simulink model "RCCA_neliniar_releu"  (R2021a)
settings: Solver=FixedStepAuto  StartTime=0.0  StopTime=20  FixedStep=0.001  RelTol=1e-6
values from neighbouring files (symbols this model uses):
  c0 = 5.4698    [initializare_model.m]
  ci = 10    [initializare_model.m]
  EdR = 49584/8.32    (= 5959.61538462)    [initializare_model.m]
  hA = kT*At    (= 18821.555234)    [initializare_model.m]
  k0 = 34930800    [initializare_model.m]
  mdH = 24953    [initializare_model.m]
  q = 10    [initializare_model.m]
  rcp = 2093    [initializare_model.m]
  T0 = 339.437    [initializare_model.m]
  Ti = 38+273    (= 311)    [initializare_model.m]
  V = 10    [initializare_model.m]
undefined symbols (not defined in the file or in its folder): kreg, tdreg, tireg, tkreg, ttdreg, ttireg
libraries: pid_lib x3
settings Model: Creator=PS  LastModifiedBy=Automatica
settings SolverCC: ZeroCrossAlgorithm=Adaptive  AlgebraicLoopSolver=TrustRegion
settings DataIOCC: ReturnWorkspaceOutputs=off
settings DebuggingCC: IgnoredZcDiagnostic=none  SFMachineParentedDataDiag=warning  ArithmeticOperatorsInVariantConditions=warning
settings SFSimCC: SimUseLocalCustomCode=off  CustomCodeUndefinedFunction=UseInterfaceOnly
settings RTWCC: RTWUseLocalCustomCode=off

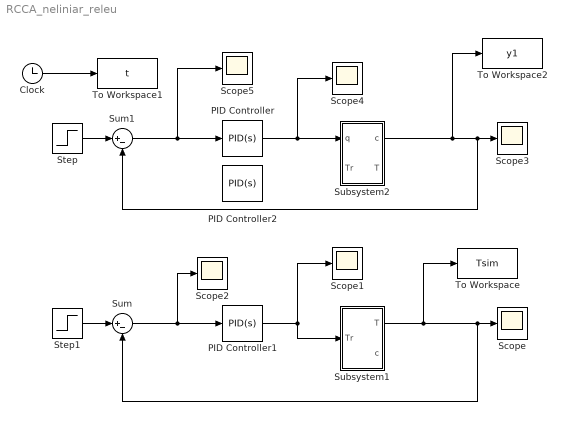
== system RCCA_neliniar_releu ==
  Clock : Clock
  PID Controller : pid_lib/PID Controller  Controller=PID  Form=Parallel  TimeDomain=Continuous-time  UseExternalTs=off  SampleTime=-1  IntegratorMethod=Forward Euler  FilterMethod=Forward Euler  ControllerParametersSource=internal  P=kreg  I=kreg/tireg  D=kreg*tdreg  UseFilter=on  N=100  TunerSelectOption=Transfer Function Based (PID Tuner App)  InitialConditionSource=internal  InitialConditionForIntegrator=q  InitialConditionForFilter=0  DifferentiatorICPrevScaledInput=0  ExternalReset=none  TrackingMode=off  Kt=1  LimitOutput=off  SatLimitsSource=internal  UpperSaturationLimit=inf  LowerSaturationLimit=-inf  LinearizeAsGain=on  AntiWindupMode=none  Kb=1  POutMin=[]  POutMax=[]  IOutMin=[]  IOutMax=[]  DOutMin=[]  DOutMax=[]  NOutMin=[]  NOutMax=[]  SumOutMin=[]  SumOutMax=[]  SaturationOutMin=[]  SaturationOutMax=[]  PParamMin=[]  PParamMax=[]  IParamMin=[]  IParamMax=[]  DParamMin=[]  DParamMax=[]  NParamMin=[]  NParamMax=[]  KbParamMin=[]  KbParamMax=[]  KtParamMin=[]  KtParamMax=[]  KbOutMin=[]  KbOutMax=[]  KtOutMin=[]  KtOutMax=[]  IntegratorOutMin=[]  IntegratorOutMax=[]  FilterOutMin=[]  FilterOutMax=[]  SumI1OutMin=[]  SumI1OutMax=[]  SumI2OutMin=[]  SumI2OutMax=[]  SumI3OutMin=[]  SumI3OutMax=[]  SumI4OutMin=[]  SumI4OutMax=[]  SumDOutMin=[]  SumDOutMax=[]  DifferentiatorOutMin=[]  DifferentiatorOutMax=[]  FilterDiffOutCoefMin=[]  FilterDiffOutCoefMax=[]  ReciprocalOutMin=[]  ReciprocalOutMax=[]  SumDenOutMin=[]  SumDenOutMax=[]  SumNumOutMin=[]  SumNumOutMax=[]  DivideOutMin=[]  DivideOutMax=[]  UdiffTsProdOutMin=[]  UdiffTsProdOutMax=[]  NTsProdOutMin=[]  NTsProdOutMax=[]  UintegralTsProdOutMin=[]  UintegralTsProdOutMax=[]  UngainTsProdOutMin=[]  UngainTsProdOutMax=[]  IntegratorContinuousStateAttributes=''  IntegratorStateMustResolveToSignalObject=off  IntegratorRTWStateStorageClass=Auto  FilterContinuousStateAttributes=''  FilterStateMustResolveToSignalObject=off  FilterRTWStateStorageClass=Auto  ParallelPVariant=InternalParameters  IdealPVariant=Disabled  IVariant=InternalParameters  DVariant=InternalParameters  IntegratorVariant=Continuous  SatVariant=Disabled  AWVariant=Passthrough  PCopyVariant=Disabled  TRVariant=Disabled  FdbkBlocksVariant=Forward  IdealPFdbkVariant=Disabled  SatFdbkVariant=Disabled  DerivativeFilterVariant=ContFilter  NVariant=InternalParameters  NCopyVariant=Disabled  FilterICVariant=InternalICsFilter  IntegratorICVariant=InternalICs  ExternalResetVariant=Disabled  TRSumVariant=Passthrough  SumFdbkVariant=Disabled  SumVariant=Sum_PID  TsampFilterVariant=InternalTs  TsampNgainVariant=Passthrough  TsampIntegralVariant=Passthrough  ExternalSaturationOutDataTypeStr=Inherit: Same as second input
  PID Controller1 : pid_lib/PID Controller  Controller=PID  Form=Parallel  TimeDomain=Continuous-time  UseExternalTs=off  SampleTime=-1  IntegratorMethod=Forward Euler  FilterMethod=Forward Euler  ControllerParametersSource=internal  P=tkreg  I=tkreg/ttireg  D=tkreg*ttdreg  UseFilter=on  N=100  TunerSelectOption=Transfer Function Based (PID Tuner App)  InitialConditionSource=internal  InitialConditionForIntegrator=Tr  InitialConditionForFilter=0  DifferentiatorICPrevScaledInput=0  ExternalReset=none  TrackingMode=off  Kt=1  LimitOutput=off  SatLimitsSource=internal  UpperSaturationLimit=inf  LowerSaturationLimit=-inf  LinearizeAsGain=on  AntiWindupMode=none  Kb=1  POutMin=[]  POutMax=[]  IOutMin=[]  IOutMax=[]  DOutMin=[]  DOutMax=[]  NOutMin=[]  NOutMax=[]  SumOutMin=[]  SumOutMax=[]  SaturationOutMin=[]  SaturationOutMax=[]  PParamMin=[]  PParamMax=[]  IParamMin=[]  IParamMax=[]  DParamMin=[]  DParamMax=[]  NParamMin=[]  NParamMax=[]  KbParamMin=[]  KbParamMax=[]  KtParamMin=[]  KtParamMax=[]  KbOutMin=[]  KbOutMax=[]  KtOutMin=[]  KtOutMax=[]  IntegratorOutMin=[]  IntegratorOutMax=[]  FilterOutMin=[]  FilterOutMax=[]  SumI1OutMin=[]  SumI1OutMax=[]  SumI2OutMin=[]  SumI2OutMax=[]  SumI3OutMin=[]  SumI3OutMax=[]  SumI4OutMin=[]  SumI4OutMax=[]  SumDOutMin=[]  SumDOutMax=[]  DifferentiatorOutMin=[]  DifferentiatorOutMax=[]  FilterDiffOutCoefMin=[]  FilterDiffOutCoefMax=[]  ReciprocalOutMin=[]  ReciprocalOutMax=[]  SumDenOutMin=[]  SumDenOutMax=[]  SumNumOutMin=[]  SumNumOutMax=[]  DivideOutMin=[]  DivideOutMax=[]  UdiffTsProdOutMin=[]  UdiffTsProdOutMax=[]  NTsProdOutMin=[]  NTsProdOutMax=[]  UintegralTsProdOutMin=[]  UintegralTsProdOutMax=[]  UngainTsProdOutMin=[]  UngainTsProdOutMax=[]  IntegratorContinuousStateAttributes=''  IntegratorStateMustResolveToSignalObject=off  IntegratorRTWStateStorageClass=Auto  FilterContinuousStateAttributes=''  FilterStateMustResolveToSignalObject=off  FilterRTWStateStorageClass=Auto  ParallelPVariant=InternalParameters  IdealPVariant=Disabled  IVariant=InternalParameters  DVariant=InternalParameters  IntegratorVariant=Continuous  SatVariant=Disabled  AWVariant=Passthrough  PCopyVariant=Disabled  TRVariant=Disabled  FdbkBlocksVariant=Forward  IdealPFdbkVariant=Disabled  SatFdbkVariant=Disabled  DerivativeFilterVariant=ContFilter  NVariant=InternalParameters  NCopyVariant=Disabled  FilterICVariant=InternalICsFilter  IntegratorICVariant=InternalICs  ExternalResetVariant=Disabled  TRSumVariant=Passthrough  SumFdbkVariant=Disabled  SumVariant=Sum_PID  TsampFilterVariant=InternalTs  TsampNgainVariant=Passthrough  TsampIntegralVariant=Passthrough  ExternalSaturationOutDataTypeStr=Inherit: Same as second input
  PID Controller2 : pid_lib/PID Controller  Controller=PID  Form=Parallel  TimeDomain=Continuous-time  UseExternalTs=off  SampleTime=-1  IntegratorMethod=Forward Euler  FilterMethod=Forward Euler  ControllerParametersSource=internal  P=tkreg  I=tkreg/ttireg  D=tkreg*ttdreg  UseFilter=on  N=100  TunerSelectOption=Transfer Function Based (PID Tuner App)  InitialConditionSource=internal  InitialConditionForIntegrator=Tr  InitialConditionForFilter=0  DifferentiatorICPrevScaledInput=0  ExternalReset=none  TrackingMode=off  Kt=1  LimitOutput=off  SatLimitsSource=internal  UpperSaturationLimit=inf  LowerSaturationLimit=-inf  LinearizeAsGain=on  AntiWindupMode=none  Kb=1  POutMin=[]  POutMax=[]  IOutMin=[]  IOutMax=[]  DOutMin=[]  DOutMax=[]  NOutMin=[]  NOutMax=[]  SumOutMin=[]  SumOutMax=[]  SaturationOutMin=[]  SaturationOutMax=[]  PParamMin=[]  PParamMax=[]  IParamMin=[]  IParamMax=[]  DParamMin=[]  DParamMax=[]  NParamMin=[]  NParamMax=[]  KbParamMin=[]  KbParamMax=[]  KtParamMin=[]  KtParamMax=[]  KbOutMin=[]  KbOutMax=[]  KtOutMin=[]  KtOutMax=[]  IntegratorOutMin=[]  IntegratorOutMax=[]  FilterOutMin=[]  FilterOutMax=[]  SumI1OutMin=[]  SumI1OutMax=[]  SumI2OutMin=[]  SumI2OutMax=[]  SumI3OutMin=[]  SumI3OutMax=[]  SumI4OutMin=[]  SumI4OutMax=[]  SumDOutMin=[]  SumDOutMax=[]  DifferentiatorOutMin=[]  DifferentiatorOutMax=[]  FilterDiffOutCoefMin=[]  FilterDiffOutCoefMax=[]  ReciprocalOutMin=[]  ReciprocalOutMax=[]  SumDenOutMin=[]  SumDenOutMax=[]  SumNumOutMin=[]  SumNumOutMax=[]  DivideOutMin=[]  DivideOutMax=[]  UdiffTsProdOutMin=[]  UdiffTsProdOutMax=[]  NTsProdOutMin=[]  NTsProdOutMax=[]  UintegralTsProdOutMin=[]  UintegralTsProdOutMax=[]  UngainTsProdOutMin=[]  UngainTsProdOutMax=[]  IntegratorContinuousStateAttributes=''  IntegratorStateMustResolveToSignalObject=off  IntegratorRTWStateStorageClass=Auto  FilterContinuousStateAttributes=''  FilterStateMustResolveToSignalObject=off  FilterRTWStateStorageClass=Auto  ParallelPVariant=InternalParameters  IdealPVariant=Disabled  IVariant=InternalParameters  DVariant=InternalParameters  IntegratorVariant=Continuous  SatVariant=Disabled  AWVariant=Passthrough  PCopyVariant=Disabled  TRVariant=Disabled  FdbkBlocksVariant=Forward  IdealPFdbkVariant=Disabled  SatFdbkVariant=Disabled  DerivativeFilterVariant=ContFilter  NVariant=InternalParameters  NCopyVariant=Disabled  FilterICVariant=InternalICsFilter  IntegratorICVariant=InternalICs  ExternalResetVariant=Disabled  TRSumVariant=Passthrough  SumFdbkVariant=Disabled  SumVariant=Sum_PID  TsampFilterVariant=InternalTs  TsampNgainVariant=Passthrough  TsampIntegralVariant=Passthrough  ExternalSaturationOutDataTypeStr=Inherit: Same as second input
  Scope{,1..5} (6 alike) : Scope
  Step : Step  Time=0  Before=c0  After=c0+0.1  SampleTime=0
  Step1 : Step  Time=0  Before=c0  After=c0+0.1  SampleTime=0
  Subsystem1 : Subsystem
  Subsystem2 : Subsystem
  Sum : Sum  Inputs=|+-  InputSameDT=on  SaturateOnIntegerOverflow=on  OutDataTypeStr=Inherit: Same as first input
  Sum1 : Sum  Inputs=|+-  InputSameDT=on  SaturateOnIntegerOverflow=on  OutDataTypeStr=Inherit: Same as first input
  To Workspace : ToWorkspace  VariableName=Tsim  SampleTime=-1
  To Workspace1 : ToWorkspace  VariableName=t  SampleTime=-1
  To Workspace2 : ToWorkspace  VariableName=y1  SampleTime=-1
  wires:
  Sum/1 -> PID Controller1/1, Scope2/1
  Step1/1 -> Sum/1
  Clock/1 -> To Workspace1/1
  Subsystem1/1("T   ") -> Scope/1, Sum/2, To Workspace/1
  Subsystem2/1(c) -> Scope3/1, Sum1/2, To Workspace2/1
  Sum1/1 -> PID Controller/1, Scope5/1
  Step/1 -> Sum1/1
  PID Controller/1 -> Scope4/1, Subsystem2/1(q)
  PID Controller1/1 -> Scope1/1, Subsystem1/1(Tr)

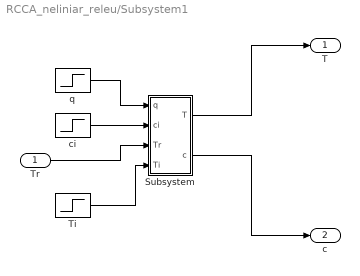
== system RCCA_neliniar_releu/Subsystem1 ==
  Tr : Inport
  Subsystem : Subsystem
  Ti : Step  Time=0  Before=Ti  After=Ti  SampleTime=0
  ci : Step  Time=0  Before=ci  After=ci  SampleTime=0
  "q  " : Step  Time=0  Before=q  After=q  SampleTime=0
  "T   " : Outport
  "c     " : Outport  Port=2
  wires:
  "q  "/1 -> Subsystem/1(q)
  ci/1 -> Subsystem/2(ci)
  Ti/1 -> Subsystem/4(Ti)
  Tr/1 -> Subsystem/3(Tr)
  Subsystem/2("c   ") -> "c     "/1
  Subsystem/1("T  ") -> "T   "/1

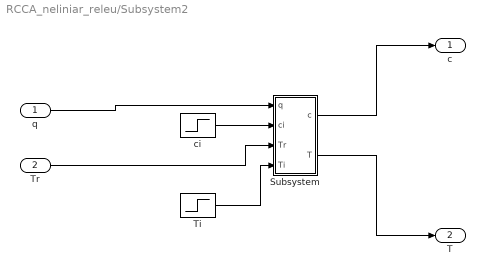
== system RCCA_neliniar_releu/Subsystem2 ==
  q : Inport
  Tr : Inport  Port=2
  Subsystem : Subsystem
  Ti : Step  Time=0  Before=Ti  After=Ti  SampleTime=0
  ci : Step  Time=0  Before=ci  After=ci  SampleTime=0
  c : Outport
  "T  " : Outport  Port=2
  wires:
  q/1 -> Subsystem/1(q)
  ci/1 -> Subsystem/2(ci)
  Ti/1 -> Subsystem/4(Ti)
  Tr/1 -> Subsystem/3(Tr)
  Subsystem/2("T  ") -> "T  "/1
  Subsystem/1(c) -> c/1

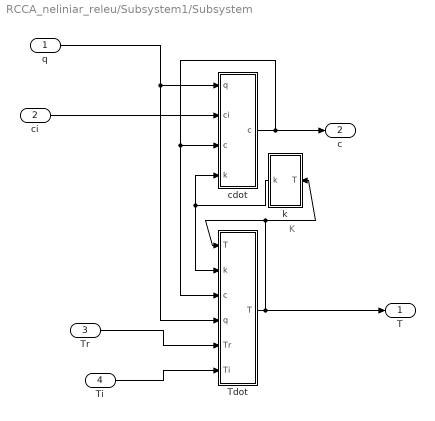
== system RCCA_neliniar_releu/Subsystem1/Subsystem ==
  note: K
  q : Inport
  ci : Inport  Port=2
  Tr : Inport  Port=3
  Ti : Inport  Port=4
  Tdot : Subsystem
  cdot : Subsystem
  k : Subsystem
  "T  " : Outport
  "c   " : Outport  Port=2
  wires:
  Tdot/1("T  ") -> "T  "/1, k/1(T), Tdot/1(T)
  k/1(k) -> Tdot/2(k), cdot/4(k)
  cdot/1(c) -> "c   "/1, cdot/3("c  "), Tdot/3(c)
  q/1 -> cdot/1(q), Tdot/4(q)
  Ti/1 -> Tdot/6(Ti)
  ci/1 -> cdot/2(ci)
  Tr/1 -> Tdot/5(Tr)

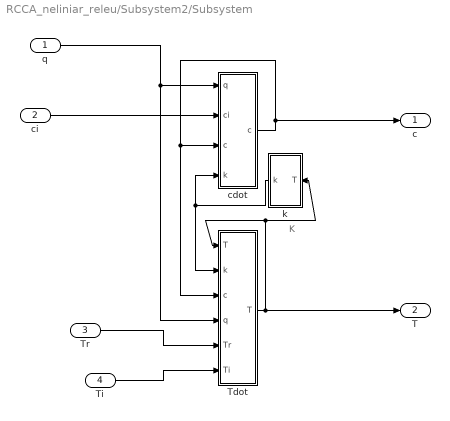
== system RCCA_neliniar_releu/Subsystem2/Subsystem ==
  note: K
  q : Inport
  ci : Inport  Port=2
  Tr : Inport  Port=3
  Ti : Inport  Port=4
  Tdot : Subsystem
  cdot : Subsystem
  k : Subsystem
  c : Outport
  "T  " : Outport  Port=2
  wires:
  Tdot/1("T  ") -> "T  "/1, k/1(T), Tdot/1(T)
  k/1(k) -> Tdot/2(k), cdot/4(k)
  cdot/1(c) -> c/1, cdot/3("c  "), Tdot/3(c)
  q/1 -> cdot/1(q), Tdot/4(q)
  Ti/1 -> Tdot/6(Ti)
  ci/1 -> cdot/2(ci)
  Tr/1 -> Tdot/5(Tr)

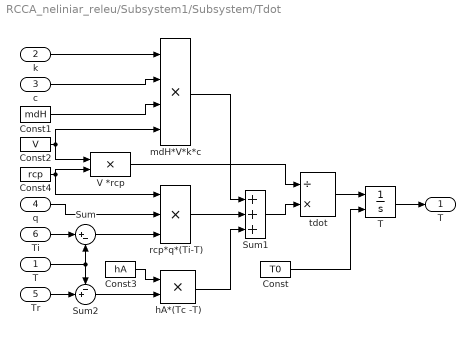
== system RCCA_neliniar_releu/Subsystem1/Subsystem/Tdot ==
  T : Inport  Interpolate=off
  k : Inport  Port=2  Interpolate=off
  c : Inport  Port=3  Interpolate=off
  q : Inport  Port=4  Interpolate=off
  Tr : Inport  Port=5  Interpolate=off
  Ti : Inport  Port=6  Interpolate=off
  Const : Constant  Value=T0
  Const1 : Constant  Value=mdH
  Const2 : Constant  Value=V
  Const3 : Constant  Value=hA
  Const4 : Constant  Value=rcp
  Sum : Sum  Inputs=|+-  InputSameDT=on  SaturateOnIntegerOverflow=on  OutDataTypeStr=Inherit: Same as first input
  Sum1 : Sum  Inputs=+++  InputSameDT=on  SaturateOnIntegerOverflow=on  OutDataTypeStr=Inherit: Same as first input
  Sum2 : Sum  Inputs=-+|  InputSameDT=on  SaturateOnIntegerOverflow=on  OutDataTypeStr=Inherit: Same as first input
  "T " : Integrator  InitialConditionSource=external
  V *rcp : Product  Inputs=**  InputSameDT=on  RndMeth=Zero  SaturateOnIntegerOverflow=on  OutDataTypeStr=Inherit: Same as first input
  hA*(Tc -T) : Product  Inputs=**  InputSameDT=on  RndMeth=Zero  SaturateOnIntegerOverflow=on  OutDataTypeStr=Inherit: Same as first input
  mdH*V*k*c : Product  Inputs=****  InputSameDT=on  RndMeth=Zero  SaturateOnIntegerOverflow=on  OutDataTypeStr=Inherit: Same as first input
  rcp*q*(Ti-T) : Product  Inputs=***  InputSameDT=on  RndMeth=Zero  SaturateOnIntegerOverflow=on  OutDataTypeStr=Inherit: Same as first input
  tdot : Product  Inputs=/*  InputSameDT=on  RndMeth=Zero  SaturateOnIntegerOverflow=on  OutDataTypeStr=Inherit: Same as first input
  "T  " : Outport
  wires:
  Ti/1 -> Sum/1
  Sum/1 -> rcp*q*(Ti-T)/3
  q/1 -> rcp*q*(Ti-T)/2
  T/1 -> Sum/2, Sum2/1
  Tr/1 -> Sum2/2
  Sum2/1 -> hA*(Tc -T)/2
  Const3/1 -> hA*(Tc -T)/1
  k/1 -> mdH*V*k*c/1
  c/1 -> mdH*V*k*c/2
  Const1/1 -> mdH*V*k*c/3
  mdH*V*k*c/1 -> Sum1/1
  rcp*q*(Ti-T)/1 -> Sum1/2
  hA*(Tc -T)/1 -> Sum1/3
  Const2/1 -> mdH*V*k*c/4, V *rcp/1
  Const4/1 -> rcp*q*(Ti-T)/1, V *rcp/2
  V *rcp/1 -> tdot/1
  Sum1/1 -> tdot/2
  tdot/1 -> "T "/1
  Const/1 -> "T "/2
  "T "/1 -> "T  "/1

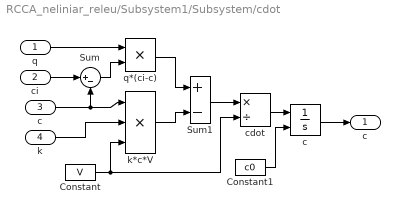
== system RCCA_neliniar_releu/Subsystem1/Subsystem/cdot ==
  q : Inport  Interpolate=off
  ci : Inport  Port=2  Interpolate=off
  "c  " : Inport  Port=3  Interpolate=off
  k : Inport  Port=4  Interpolate=off
  Constant : Constant  Value=V
  Constant1 : Constant  Value=c0
  Sum : Sum  Inputs=|+-  InputSameDT=on  SaturateOnIntegerOverflow=on  OutDataTypeStr=Inherit: Same as first input
  Sum1 : Sum  Inputs=+-  InputSameDT=on  SaturateOnIntegerOverflow=on  OutDataTypeStr=Inherit: Same as first input
  "c " : Integrator  InitialConditionSource=external
  cdot : Product  Inputs=*/  InputSameDT=on  RndMeth=Zero  SaturateOnIntegerOverflow=on  OutDataTypeStr=Inherit: Same as first input
  k*c*V : Product  Inputs=***  InputSameDT=on  RndMeth=Zero  SaturateOnIntegerOverflow=on  OutDataTypeStr=Inherit: Same as first input
  q*(ci-c) : Product  Inputs=**  InputSameDT=on  RndMeth=Zero  SaturateOnIntegerOverflow=on  OutDataTypeStr=Inherit: Same as first input
  c : Outport
  wires:
  ci/1 -> Sum/1
  "c  "/1 -> k*c*V/1, Sum/2
  q/1 -> q*(ci-c)/1
  Sum/1 -> q*(ci-c)/2
  k/1 -> k*c*V/2
  q*(ci-c)/1 -> Sum1/1
  k*c*V/1 -> Sum1/2
  Sum1/1 -> cdot/1
  Constant/1 -> k*c*V/3, cdot/2
  cdot/1 -> "c "/1
  "c "/1 -> c/1
  Constant1/1 -> "c "/2

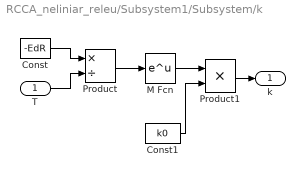
== system RCCA_neliniar_releu/Subsystem1/Subsystem/k ==
  T : Inport  Interpolate=off
  Const : Constant  Value=-EdR
  Const1 : Constant  Value=k0
  M Fcn : Math  SignedPower=on  SaturateOnIntegerOverflow=on
  Product : Product  Inputs=*/  InputSameDT=on  RndMeth=Zero  SaturateOnIntegerOverflow=on  OutDataTypeStr=Inherit: Same as first input
  Product1 : Product  Inputs=**  InputSameDT=on  RndMeth=Zero  SaturateOnIntegerOverflow=on  OutDataTypeStr=Inherit: Same as first input
  k : Outport
  wires:
  Const/1 -> Product/1
  T/1 -> Product/2
  Product/1 -> M Fcn/1
  M Fcn/1 -> Product1/1
  Const1/1 -> Product1/2
  Product1/1 -> k/1

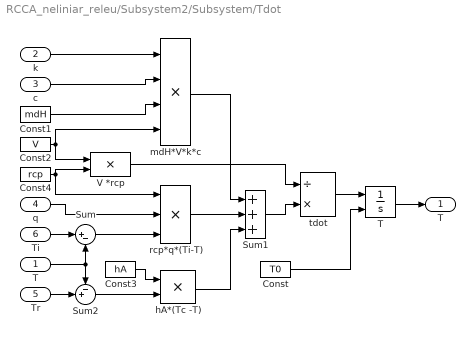
== system RCCA_neliniar_releu/Subsystem2/Subsystem/Tdot ==
  T : Inport  Interpolate=off
  k : Inport  Port=2  Interpolate=off
  c : Inport  Port=3  Interpolate=off
  q : Inport  Port=4  Interpolate=off
  Tr : Inport  Port=5  Interpolate=off
  Ti : Inport  Port=6  Interpolate=off
  Const : Constant  Value=T0
  Const1 : Constant  Value=mdH
  Const2 : Constant  Value=V
  Const3 : Constant  Value=hA
  Const4 : Constant  Value=rcp
  Sum : Sum  Inputs=|+-  InputSameDT=on  SaturateOnIntegerOverflow=on  OutDataTypeStr=Inherit: Same as first input
  Sum1 : Sum  Inputs=+++  InputSameDT=on  SaturateOnIntegerOverflow=on  OutDataTypeStr=Inherit: Same as first input
  Sum2 : Sum  Inputs=-+|  InputSameDT=on  SaturateOnIntegerOverflow=on  OutDataTypeStr=Inherit: Same as first input
  "T " : Integrator  InitialConditionSource=external
  V *rcp : Product  Inputs=**  InputSameDT=on  RndMeth=Zero  SaturateOnIntegerOverflow=on  OutDataTypeStr=Inherit: Same as first input
  hA*(Tc -T) : Product  Inputs=**  InputSameDT=on  RndMeth=Zero  SaturateOnIntegerOverflow=on  OutDataTypeStr=Inherit: Same as first input
  mdH*V*k*c : Product  Inputs=****  InputSameDT=on  RndMeth=Zero  SaturateOnIntegerOverflow=on  OutDataTypeStr=Inherit: Same as first input
  rcp*q*(Ti-T) : Product  Inputs=***  InputSameDT=on  RndMeth=Zero  SaturateOnIntegerOverflow=on  OutDataTypeStr=Inherit: Same as first input
  tdot : Product  Inputs=/*  InputSameDT=on  RndMeth=Zero  SaturateOnIntegerOverflow=on  OutDataTypeStr=Inherit: Same as first input
  "T  " : Outport
  wires:
  Ti/1 -> Sum/1
  Sum/1 -> rcp*q*(Ti-T)/3
  q/1 -> rcp*q*(Ti-T)/2
  T/1 -> Sum/2, Sum2/1
  Tr/1 -> Sum2/2
  Sum2/1 -> hA*(Tc -T)/2
  Const3/1 -> hA*(Tc -T)/1
  k/1 -> mdH*V*k*c/1
  c/1 -> mdH*V*k*c/2
  Const1/1 -> mdH*V*k*c/3
  mdH*V*k*c/1 -> Sum1/1
  rcp*q*(Ti-T)/1 -> Sum1/2
  hA*(Tc -T)/1 -> Sum1/3
  Const2/1 -> mdH*V*k*c/4, V *rcp/1
  Const4/1 -> rcp*q*(Ti-T)/1, V *rcp/2
  V *rcp/1 -> tdot/1
  Sum1/1 -> tdot/2
  tdot/1 -> "T "/1
  Const/1 -> "T "/2
  "T "/1 -> "T  "/1

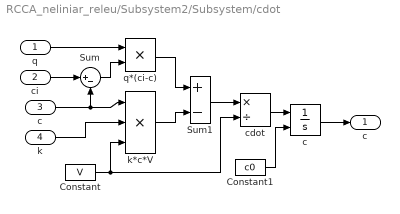
== system RCCA_neliniar_releu/Subsystem2/Subsystem/cdot ==
  q : Inport  Interpolate=off
  ci : Inport  Port=2  Interpolate=off
  "c  " : Inport  Port=3  Interpolate=off
  k : Inport  Port=4  Interpolate=off
  Constant : Constant  Value=V
  Constant1 : Constant  Value=c0
  Sum : Sum  Inputs=|+-  InputSameDT=on  SaturateOnIntegerOverflow=on  OutDataTypeStr=Inherit: Same as first input
  Sum1 : Sum  Inputs=+-  InputSameDT=on  SaturateOnIntegerOverflow=on  OutDataTypeStr=Inherit: Same as first input
  "c " : Integrator  InitialConditionSource=external
  cdot : Product  Inputs=*/  InputSameDT=on  RndMeth=Zero  SaturateOnIntegerOverflow=on  OutDataTypeStr=Inherit: Same as first input
  k*c*V : Product  Inputs=***  InputSameDT=on  RndMeth=Zero  SaturateOnIntegerOverflow=on  OutDataTypeStr=Inherit: Same as first input
  q*(ci-c) : Product  Inputs=**  InputSameDT=on  RndMeth=Zero  SaturateOnIntegerOverflow=on  OutDataTypeStr=Inherit: Same as first input
  c : Outport
  wires:
  ci/1 -> Sum/1
  "c  "/1 -> k*c*V/1, Sum/2
  q/1 -> q*(ci-c)/1
  Sum/1 -> q*(ci-c)/2
  k/1 -> k*c*V/2
  q*(ci-c)/1 -> Sum1/1
  k*c*V/1 -> Sum1/2
  Sum1/1 -> cdot/1
  Constant/1 -> k*c*V/3, cdot/2
  cdot/1 -> "c "/1
  "c "/1 -> c/1
  Constant1/1 -> "c "/2

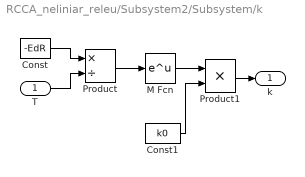
== system RCCA_neliniar_releu/Subsystem2/Subsystem/k ==
  T : Inport  Interpolate=off
  Const : Constant  Value=-EdR
  Const1 : Constant  Value=k0
  M Fcn : Math  SignedPower=on  SaturateOnIntegerOverflow=on
  Product : Product  Inputs=*/  InputSameDT=on  RndMeth=Zero  SaturateOnIntegerOverflow=on  OutDataTypeStr=Inherit: Same as first input
  Product1 : Product  Inputs=**  InputSameDT=on  RndMeth=Zero  SaturateOnIntegerOverflow=on  OutDataTypeStr=Inherit: Same as first input
  k : Outport
  wires:
  Const/1 -> Product/1
  T/1 -> Product/2
  Product/1 -> M Fcn/1
  M Fcn/1 -> Product1/1
  Const1/1 -> Product1/2
  Product1/1 -> k/1
